simulink model "NFO"  (R2023a)
settings: Solver=FixedStepDiscrete  StartTime=0.0  StopTime=10  FixedStep=TsModel  RelTol=1e-3
values from neighbouring files (symbols this model uses):
  ADRC_times = 1.0    [NFO.sldd]
  b0 = 10000.0    [NFO.sldd]
  CCR_Counter = 8000.0    [NFO.sldd]
  current_bandwidth = 1500.0    [NFO.sldd]
  FLL_K = 1.414    [NFO.sldd]
  flux = 0.011    [NFO.sldd]
  Idq_limit = 20.0    [NFO.sldd]
  IF_Initial = 40.0    [NFO.sldd]
  Ls = 0.0001952    [NFO.sldd]
  Min_FLL_omega = 10.0    [NFO.sldd]
  omega_c = 50.0    [NFO.sldd]
  PLL_I = 3000.0    [NFO.sldd]
  PLL_P = 10.0    [NFO.sldd]
  PMSM_B = 0.0004924    [NFO.sldd]
  PMSM_J = 0.0027    [NFO.sldd]
  PMSM_Pn = 5.0    [NFO.sldd]
  Pn = 5.0    [NFO.sldd]
  Rs = 0.1763    [NFO.sldd]
  Swich_time = 1.5    [NFO.sldd]
  tao = -30.0    [NFO.sldd]
  Ts = 0.0001    [NFO.sldd]
  TsModel = 2.5E-5    [NFO.sldd]
undefined symbols (not defined in the file or in its folder): DiscIntNeverNeededParam, sigbuilder_block
libraries: slpidlib x3, mcbplantlib x1, autolibpmsmexterior x1
(part 1 of 2)
settings Model: DataDictionary=NFO.sldd  Creator=33595  LastModifiedBy=SkyLin
settings OptimizationCC: DefaultParameterBehavior=Inlined  UseDivisionForNetSlopeComputation=on  GainParamInheritBuiltInType=on  UseFloatMulNetSlope=on  InlineInvariantSignals=on  PassReuseOutputArgsAs=Individual arguments  ZeroExternalMemoryAtStartup=off  ZeroInternalMemoryAtStartup=off  NoFixptDivByZeroProtection=on  EfficientFloat2IntCast=on  LifeSpan=1  OptimizeBlockOrder=speed  DifferentSizesBufferReuse=on  EfficientTunableParamExpr=on
settings DebuggingCC: ParameterOverflowMsg=none  ParameterUnderflowMsg=error  ParameterPrecisionLossMsg=none  ParameterTunabilityLossMsg=error  UnconnectedInputMsg=warning  UnconnectedOutputMsg=warning  UnconnectedLineMsg=warning
settings HardwareCC: ProdBitPerPointer=32  ProdBitPerSizeT=32  ProdBitPerPtrDiffT=32  ProdLargestAtomicInteger=Long  ProdLargestAtomicFloat=Double  ProdWordSize=32  ProdLongLongMode=on  ProdHWDeviceType=ARM Compatible->ARM Cortex-M
settings ModelReferenceCC: EnableRefExpFcnMdlSchedulingChecks=on
settings SFSimCC: MATLABDynamicMemAlloc=off
settings RTWCC: Description=Embedded Coder  SystemTargetFile=ert.tlc  GenCodeOnly=on  TemplateMakefile=ert_default_tmf  RTWUseSimCustomCode=on  DLArmComputeVersion=19.05
settings CodeAppCC: ForceParamTrailComments=on  IgnoreCustomStorageClasses=off  OperatorAnnotations=on  SimulinkDataObjDesc=on  SFDataObjDesc=on  CustomSymbolStrGlobalVar=rt$N$M  CustomSymbolStrType=$N$M  CustomSymbolStrFcn=$N$M$F  CustomSymbolStrMacro=$N$M  InsertBlockDesc=on
settings ERTTargetCC: TargetLangStandard=C99 (ISO)  CodeReplacementLibrary=ARM Cortex-M  GenerateSampleERTMain=on  IncludeMdlTerminateFcn=off  CombineSignalStateStructs=on  SupportComplex=off  SupportNonInlinedSFcns=on  InlinedParameterPlacement=NonHierarchical  ERTCustomFileTemplate=example_file_process.tlc  ERTFilePackagingFormat=CompactWithDataFile  IndentSize=4

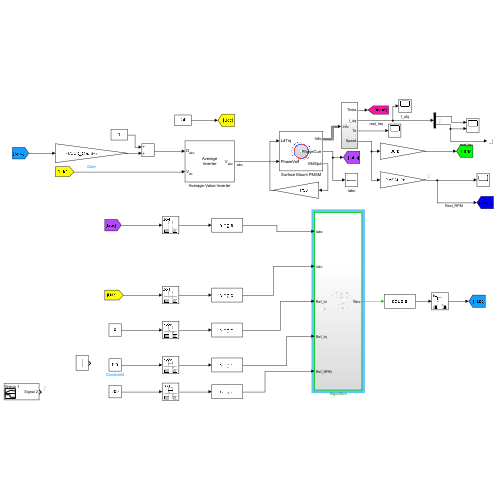
[thumbnail: Simulink's stored preview of the top-level diagram]
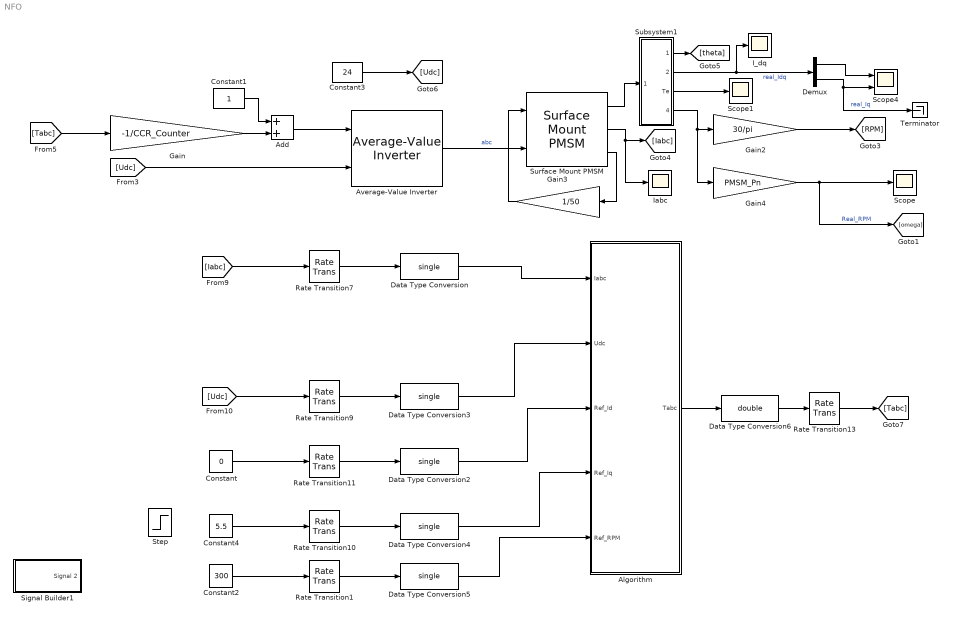
== system NFO ==
  Add : Sum
  Algorithm : Subsystem  TreatAsAtomicUnit=on
  Average-Value Inverter : mcbplantlib/Average-Value Inverter
  Constant : Constant  Value=0  OutDataTypeStr=single  SampleTime=Ts
  Constant1 : Constant  SampleTime=TsModel
  Constant2 : Constant  Value=300
  Constant3 : Constant  Value=24  SampleTime=TsModel
  Constant4 : Constant  Value=5.5  OutDataTypeStr=single  SampleTime=Ts
  Data Type Conversion{,2..5} (5 alike) : DataTypeConversion  OutDataTypeStr=single  SaturateOnIntegerOverflow=off  RndMeth=Floor
  Data Type Conversion6 : DataTypeConversion  OutDataTypeStr=double  SaturateOnIntegerOverflow=off  RndMeth=Floor
  Demux : Demux  Outputs=2
  Gain : Gain  Gain=-1/CCR_Counter
  Gain2 : Gain  Gain=30/pi
  Gain3 : Gain  Gain=1/50
  Gain4 : Gain  Gain=PMSM_Pn
  I_dq : Scope
  Iabc : Scope
  Rate Transition{1,9..11} (4 alike) : RateTransition  OutPortSampleTime=Ts
  Rate Transition13 : RateTransition  OutPortSampleTime=TsModel
  Rate Transition7 : RateTransition
  Scope : Scope
  Scope1 : Scope
  Scope4 : Scope  NumInputPorts=2
  Signal Builder1 : Subsystem  Tag=STV Subsys  LoadFcn=sigbuilder_block('load');  StartFcn=sigbuilder_block('start');  StopFcn=sigbuilder_block('stop');  ClipboardFcn=sigbuilder_block('clipboard');  mask(Sigbuilder block){tuvar=[0:10]}
      mask help: Simulink:masks:SigbuilderBlock_MD
      mask init:
      | if ~strcmp(get_param(bdroot(gcbh),'SimulationStatus'),'stopped') tuvar = sigbuilder_block('maskInit'); end
      settings: CopyFcn=sigbuilder_block('copy');  DeleteFcn=sigbuilder_block('delete');  ModelCloseFcn=sigbuilder_block('modelClose');  PreSaveFcn=sigbuilder_block('preSave');  PauseFcn=sigbuilder_block('pause');  ContinueFcn=sigbuilder_block('continue');  NameChangeFcn=sigbuilder_block('namechange');  OpenFcn=sigbuilder_block('open',[604 168 670.5 300 ]);  CloseFcn=sigbuilder_block('close');
      mask Display: plot(0, 0, 100, 100,[2, 2, 32, 32, 2], [68, 8, 8, 68, 68],[32, 2], [38, 38], [32, 19, 2],[53, 60, 44], [32, 17, 17, 2],[16, 16, 31, 31]);txt = getActiveGroup(gcbh);text(2, 100, txt,'verticalAlignment', 'top');
  Step : Step  Time=0  After=10  SampleTime=TsModel
  Subsystem1 : Subsystem
  Surface Mount PMSM : autolibpmsmexterior/Surface Mount PMSM  port_config=Torque  sim_type=Discrete  Ts=TsModel  P=PMSM_Pn  Rs=PMSM_Rs  Ldq_=PMSM_Ls  KConstText=Permanent flux linkage constant (lambda_pm):  lambda_pm=PMSM_flux  Ke=159.9771  Kt=1.323  mechanical=[PMSM_J, PMSM_B, 0]  idq0=[0 0]  theta_init=1  omega_init=0  KConst=PMSM_flux  lambda_pm_calc=PMSM_flux  RefBlkName='autolibpmsmexterior/Surface Mount PMSM'  aMode=5  Ldq="[0.0017      0.0017]"
  Terminator : Terminator
  wires:
  Constant3/1 -> [Udc]
  [Tabc] -> Gain/1
  Subsystem1/1(Theta) -> [theta]
  Subsystem1/2(I_dq) -> Demux/1, I_dq/1  "real_Idq"
  Subsystem1/3(Te) -> Scope1/1
  Subsystem1/4(Speed) -> Gain4/1, Gain2/1
  Average-Value Inverter/1 -> Surface Mount PMSM/2  "abc"
  Surface Mount PMSM/1 -> Subsystem1/1(Info)
  Surface Mount PMSM/2 -> Iabc/1, [Iabc]
  [Udc] -> Average-Value Inverter/2
  Gain2/1 -> [RPM]
  Surface Mount PMSM/3 -> Gain3/1
  Gain3/1 -> Surface Mount PMSM/1
  Gain4/1 -> [omega], Scope/1  "Real_RPM"
  Demux/2 -> Scope4/2, Terminator/1  "real_Iq"
  Data Type Conversion2/1 -> Algorithm/3(Ref_Id)
  [Udc] -> Rate Transition9/1
  Rate Transition13/1 -> [Tabc]
  [Iabc] -> Rate Transition7/1
  Rate Transition10/1 -> Data Type Conversion4/1
  Algorithm/1(Tabc) -> Data Type Conversion6/1
  Data Type Conversion/1 -> Algorithm/1(Iabc)
  Rate Transition11/1 -> Data Type Conversion2/1
  Rate Transition7/1 -> Data Type Conversion/1
  Data Type Conversion6/1 -> Rate Transition13/1
  Constant/1 -> Rate Transition11/1
  Data Type Conversion4/1 -> Algorithm/4(Ref_Iq)
  Rate Transition9/1 -> Data Type Conversion3/1
  Data Type Conversion3/1 -> Algorithm/2(Udc)
  Add/1 -> Average-Value Inverter/1
  Gain/1 -> Add/2
  Constant1/1 -> Add/1
  Demux/1 -> Scope4/1
  Rate Transition1/1 -> Data Type Conversion5/1
  Data Type Conversion5/1 -> Algorithm/5(Ref_RPM)
  Constant2/1 -> Rate Transition1/1
  Constant4/1 -> Rate Transition10/1

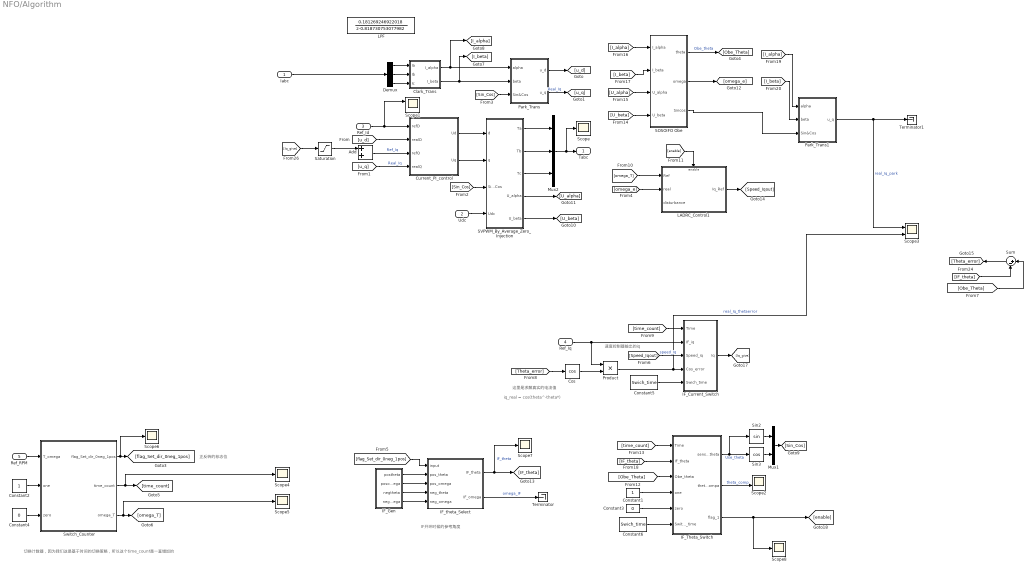
== system NFO/Algorithm ==
  note: iq_real = cos(theta^-theta*)
  note: 这里是求解真实的电流值
  note: 速度控制器输出的iq
  note: 正反转的标志位
  note: IF开环时候的参考角度
  note: 切换计数器，因为我们这是基于时间的切换策略，所以这个time_count是一直增加的
  Iabc : Inport  OutDataTypeStr=single
  Udc : Inport  Port=2  OutDataTypeStr=single
  Ref_Id : Inport  Port=3  OutDataTypeStr=single
  Ref_Iq : Inport  Port=4  OutDataTypeStr=single
  Ref_RPM : Inport  Port=5
  " Switch_Counter" : MATLAB Function  TreatAsAtomicUnit=on
  Add : Sum  OutDataTypeStr=single
  Clark_Trans : Subsystem  TreatAsAtomicUnit=on
      settings: RTWFcnNameOpts=Use subsystem name
  Constant1 : Constant  OutDataTypeStr=single
  Constant2 : Constant  OutDataTypeStr=single
  Constant3 : Constant  Value=0  OutDataTypeStr=single
  Constant4 : Constant  Value=0  OutDataTypeStr=single
  Constant5 : Constant  Value=Swich_time  OutDataTypeStr=single
  Constant6 : Constant  Value=Swich_time  OutDataTypeStr=single
  Cos : Trigonometry  Operator=cos
  Current_PI_control : Subsystem  TreatAsAtomicUnit=on
      settings: RTWFcnNameOpts=Use subsystem name
  Demux : Demux  Outputs=3
  IF_Current_Switch : MATLAB Function  TreatAsAtomicUnit=on
  IF_Gen : Subsystem
  IF_Theta_Switch : MATLAB Function  TreatAsAtomicUnit=on
  IF_theta_Select : MATLAB Function  TreatAsAtomicUnit=on
  LADRC_Control1 : Subsystem  TreatAsAtomicUnit=on
  LPF : DiscreteTransferFcn  Numerator=[0.181269246922018]  Denominator=[1 -0.818730753077982]
  Mux1 : Mux  Inputs=2
  Mux2 : Mux  Inputs=3
  Park_Trans : Subsystem  TreatAsAtomicUnit=on
      settings: RTWFcnNameOpts=Use subsystem name
  Park_Trans1 : Subsystem  TreatAsAtomicUnit=on
      settings: RTWFcnNameOpts=Use subsystem name
  Product : Product
  SOSOIFO Obe : Subsystem
  SVPWM_By_Average_Zero_Injection : Subsystem  TreatAsAtomicUnit=on
  Saturation : Saturate  UpperLimit=Idq_limit  LowerLimit=-Idq_limit  OutDataTypeStr=single
  Scope{,4..8} (6 alike) : Scope
  Scope1 : Scope  NumInputPorts=2
  Scope2 : Scope  NumInputPorts=2
  Scope3 : Scope  NumInputPorts=2
  Sin2 : Trigonometry
  Sin3 : Trigonometry  Operator=cos
  Sum : Sum  Inputs=|+-
  Terminator : Terminator
  Terminator1 : Terminator
  Tabc : Outport  OutDataTypeStr=single
  wires:
  Clark_Trans/2(I_beta) -> [I_beta], Park_Trans/2(beta)
  Clark_Trans/1(I_alpha) -> [I_alpha], Park_Trans/1(alpha)
  Demux/1 -> Clark_Trans/1(Ia)
  Demux/2 -> Clark_Trans/2(Ib)
  Demux/3 -> Clark_Trans/3(Ic)
  Park_Trans/1(u_d) -> [u_d]
  Park_Trans/2(u_q) -> [u_q]  "Real_Iq"
  Udc/1 -> SVPWM_By_Average_Zero_Injection/4(Udc)
  SVPWM_By_Average_Zero_Injection/1(Ta) -> Mux2/1
  SVPWM_By_Average_Zero_Injection/2(Tb) -> Mux2/2
  SVPWM_By_Average_Zero_Injection/3(Tc) -> Mux2/3
  SVPWM_By_Average_Zero_Injection/4(U_alpha) -> [U_alpha]
  SVPWM_By_Average_Zero_Injection/5(U_beta) -> [U_beta]
  [u_d] -> Current_PI_control/2(realD)
  [u_q] -> Current_PI_control/4(realQ)  "Real_Iq"
  Current_PI_control/1(Ud) -> SVPWM_By_Average_Zero_Injection/1(d)
  Current_PI_control/2(Uq) -> SVPWM_By_Average_Zero_Injection/2(q)
  [Sin_Cos] -> SVPWM_By_Average_Zero_Injection/3(Sin&Cos)
  [Sin_Cos] -> Park_Trans/3(Sin&Cos)
  Mux2/1 -> Tabc/1, Scope/1
  SOSOIFO Obe/1(theta) -> [Obe_Theta]  "Obe_theta"
  SOSOIFO Obe/2(omega) -> [omega_e]
  [I_alpha] -> SOSOIFO Obe/1(I_alpha)
  [U_alpha] -> SOSOIFO Obe/3(U_alpha)
  [I_beta] -> SOSOIFO Obe/2(I_beta)
  [U_beta] -> SOSOIFO Obe/4(U_beta)
  Ref_Id/1 -> Scope1/1, Current_PI_control/1(refD)
  [omega_e] -> LADRC_Control1/2(real)
  [omega_T] -> LADRC_Control1/1(Ref)
  Iabc/1 -> Demux/1
  Add/1 -> Current_PI_control/3(refQ)  "Ref_Iq"
  Constant2/1 -> " Switch_Counter"/2(one)
  Constant4/1 -> " Switch_Counter"/3(zero)
  Ref_RPM/1 -> " Switch_Counter"/1(T_omega)
  " Switch_Counter"/2(time_count) -> Scope4/1, [time_count]
  " Switch_Counter"/3(omega_T) -> Scope5/1, [omega_T]
  [Iq_give] -> Saturation/1
  Sum/1 -> [Theta_error]
  [Theta_error] -> Cos/1
  [Obe_Theta] -> Sum/1
  Constant3/1 -> IF_Theta_Switch/5(zero)
  IF_Theta_Switch/3(flag_1) -> Scope8/1, [enable]
  [IF_theta] -> Sum/2
  IF_Theta_Switch/1(sensorless_theta) -> Sin2/1, Sin3/1  "Use_theta"
  Sin3/1 -> Mux1/2
  Sin2/1 -> Mux1/1
  IF_Current_Switch/1(Iq) -> [Iq_give]
  Constant1/1 -> IF_Theta_Switch/4(one)
  LADRC_Control1/1(Iq_Ref) -> [Speed_Iqout]
  Ref_Iq/1 -> Product/1, IF_Current_Switch/2(IF_iq)
  [enable] -> LADRC_Control1/Enable
  " Switch_Counter"/1(flag_Set_dir_0neg_1pos) -> Scope6/1, [flag_Set_dir_0neg_1pos]
  Mux1/1 -> [Sin_Cos]
  Saturation/1 -> Add/1
  IF_Gen/1(postheta) -> IF_theta_Select/2(pos_theta)
  IF_Gen/2(posomega) -> IF_theta_Select/3(pos_omega)
  IF_Gen/3(negtheta) -> IF_theta_Select/4(neg_theta)
  IF_Gen/4(negomega) -> IF_theta_Select/5(neg_omega)
  [flag_Set_dir_0neg_1pos] -> IF_theta_Select/1(input)
  IF_theta_Select/1(IF_theta) -> Scope7/1, [IF_theta]  "IF_theta"
  [Obe_Theta] -> IF_Theta_Switch/3(Obe_theta)
  IF_Theta_Switch/2(theta_compa) -> Scope2/2  "theta_comp"
  [time_count] -> IF_Current_Switch/1(Time)
  [time_count] -> IF_Theta_Switch/1(Time)
  [Speed_Iqout] -> IF_Current_Switch/3(Speed_iq)  "speed_Iq"
  Product/1 -> Scope3/2, IF_Current_Switch/4(Cos_error)  "real_Iq_thetaerror"
  Cos/1 -> Product/2
  Constant5/1 -> IF_Current_Switch/5(Swich_time)
  IF_theta_Select/2(IF_omega) -> Terminator/1  "omega_IF"
  Constant6/1 -> IF_Theta_Switch/6(Switch_time)
  [IF_theta] -> IF_Theta_Switch/2(IF_theta)
  SOSOIFO Obe/3(Sincos) -> Park_Trans1/3(Sin&Cos)
  [I_beta] -> Park_Trans1/2(beta)
  [I_alpha] -> Park_Trans1/1(alpha)
  Park_Trans1/1(u_q) -> Scope3/1, Terminator1/1  "real_Iq_park"

== system NFO/Signal Builder1 ==
  Demux : Demux  Tag=STV Demux  Outputs=1
      settings: DisplayOption=none
  FromWs : FromWorkspace  Tag=STV FromWs  VariableName=tuvar
      SigBuilderData=|
      | common.afterFinalStr = 'Extrapolate'
      | common.sampleTime = 0
      | dataSet.timeRange = [0 10]
      | dataSet.name = 'Group 1'
      | sbobj.Groups.Name = 'Group 1'
      | sbobj.Groups.Signals.Name = 'Signal 2'
      | sbobj.Groups.Signals.XData = [0 5.72 5.72 10]
      | sbobj.Groups.Signals.YData = [126 126 234 234]
  Signal 2 : Outport  Tag=STV Outport
  wires:
  Demux/1 -> Signal 2/1
  FromWs/1 -> Demux/1

== system NFO/Subsystem1 ==
  Info : Inport
  Bus Selector2 : BusSelector  OutputSignals=IdSync,IqSync,MtrPos,MtrTrq,MtrSpd
  Constant4 : Constant  Value=2*pi  SampleTime=-1
  Gain2 : Gain  Gain=Pn
  Mod1 : Math  Operator=mod
  Mux : Mux  Inputs=2
  Scope : Scope
  Theta : Outport
  I_dq : Outport  Port=2
  Te : Outport  Port=3
  Speed : Outport  Port=4
  wires:
  Bus Selector2/2 -> Mux/2  "<IqSync>"
  Gain2/1 -> Mod1/1
  Mod1/1 -> Theta/1
  Bus Selector2/1 -> Mux/1  "<IdSync>"
  Constant4/1 -> Mod1/2
  Info/1 -> Bus Selector2/1
  Bus Selector2/3 -> Gain2/1  "<MtrPos>"
  Mux/1 -> I_dq/1
  Bus Selector2/4 -> Te/1  "<MtrTrq>"
  Bus Selector2/5 -> Scope/1, Speed/1  "<MtrSpd>"

== system NFO/Algorithm/Clark_Trans ==
  note: $u_\alpha=\frac{2}{3}(u_a-\frac{1}{2}u_b-\frac{1}{2}u_c ) \\ u_\beta=\frac{2}{3}(\frac{\sqrt{3}}{2}u_b-\frac{\sqrt{3}}{2}u_c)$
  note: Clark_Transform
  Ia : Inport  OutDataTypeStr=single
  Ib : Inport  Port=2  OutDataTypeStr=single
  Ic : Inport  Port=3  OutDataTypeStr=single
  Add : Sum  Inputs=+-  OutDataTypeStr=single
  Add1 : Sum  OutDataTypeStr=single
  Add2 : Sum  Inputs=+-  OutDataTypeStr=single
  Gain : Gain  Gain=0.5  OutDataTypeStr=single
  Gain1 : Gain  Gain=single(sqrt(3)/3)  OutDataTypeStr=single
  Gain2 : Gain  Gain=single(2/3)  OutDataTypeStr=single
  I_alpha : Outport  OutDataTypeStr=single
  I_beta : Outport  Port=2
  wires:
  Ia/1 -> Add/1
  Gain/1 -> Add/2
  Ib/1 -> Add1/1, Add2/1
  Ic/1 -> Add1/2, Add2/2
  Add2/1 -> Gain1/1
  Add1/1 -> Gain/1
  Add/1 -> Gain2/1
  Gain2/1 -> I_alpha/1
  Gain1/1 -> I_beta/1

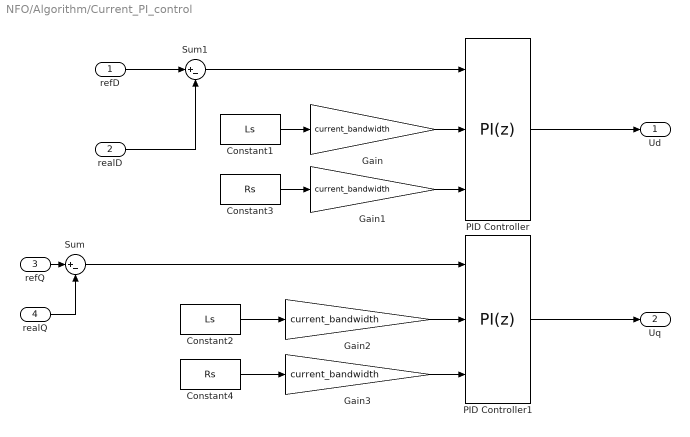
== system NFO/Algorithm/Current_PI_control ==
  refD : Inport  OutDataTypeStr=single
  realD : Inport  Port=2  OutDataTypeStr=single
  refQ : Inport  Port=3  OutDataTypeStr=single
  realQ : Inport  Port=4  OutDataTypeStr=single
  Constant1 : Constant  Value=Ls  OutDataTypeStr=single  SampleTime=Ts
  Constant2 : Constant  Value=Ls  OutDataTypeStr=single  SampleTime=Ts
  Constant3 : Constant  Value=Rs  OutDataTypeStr=single  SampleTime=Ts
  Constant4 : Constant  Value=Rs  OutDataTypeStr=single  SampleTime=Ts
  Gain{,1..3} (4 alike) : Gain  Gain=current_bandwidth  OutDataTypeStr=single
  PID Controller : slpidlib/PID Controller  Controller=PI  Form=Parallel  TimeDomain=Discrete-time  UseExternalTs=off  SampleTime=Ts  IntegratorMethod=Forward Euler  FilterMethod=Forward Euler  ControllerParametersSource=external  P=1  I=1  UseKiTs=off  D=0  N=100  UseFilter=on  TunerSelectOption=Transfer Function Based (PID Tuner App)  ZeroCross=off  InitialConditionSource=internal  InitialConditionForIntegrator=0  InitialConditionForFilter=0  DifferentiatorICPrevScaledInput=0  ExternalReset=none  TrackingMode=off  Kt=1  LimitOutput=on  SatLimitsSource=internal  UpperSaturationLimit=Idq_limit  LowerSaturationLimit=-Idq_limit  LinearizeAsGain=off  AntiWindupMode=none  Kb=1  LimitIntegrator=off  UpperIntegratorSaturationLimit=inf  LowerIntegratorSaturationLimit=-inf  POutMin=[]  POutMax=[]  IOutMin=[]  IOutMax=[]  DOutMin=[]  DOutMax=[]  NOutMin=[]  NOutMax=[]  SumOutMin=[]  SumOutMax=[]  SaturationOutMin=[]  SaturationOutMax=[]  PParamMin=[]  PParamMax=[]  IParamMin=[]  IParamMax=[]  DParamMin=[]  DParamMax=[]  NParamMin=[]  NParamMax=[]  KbParamMin=[]  KbParamMax=[]  KtParamMin=[]  KtParamMax=[]  KbOutMin=[]  KbOutMax=[]  KtOutMin=[]  KtOutMax=[]  IntegratorOutMin=[]  IntegratorOutMax=[]  FilterOutMin=[]  FilterOutMax=[]  SumI1OutMin=[]  SumI1OutMax=[]  SumI2OutMin=[]  SumI2OutMax=[]  SumI3OutMin=[]  SumI3OutMax=[]  SumI4OutMin=[]  SumI4OutMax=[]  SumDOutMin=[]  SumDOutMax=[]  DifferentiatorOutMin=[]  DifferentiatorOutMax=[]  FilterDiffOutCoefMin=[]  FilterDiffOutCoefMax=[]  ReciprocalOutMin=[]  ReciprocalOutMax=[]  SumDenOutMin=[]  SumDenOutMax=[]  SumNumOutMin=[]  SumNumOutMax=[]  DivideOutMin=[]  DivideOutMax=[]  UdiffTsProdOutMin=[]  UdiffTsProdOutMax=[]  NTsProdOutMin=[]  NTsProdOutMax=[]  UintegralTsProdOutMin=[]  UintegralTsProdOutMax=[]  UngainTsProdOutMin=[]  UngainTsProdOutMax=[]  ClampingZeroOutDataTypeStr=Inherit: Inherit via back propagation  ClampingZeroOutMin=[]  ClampingZeroOutMax=[]  FilterDenConstantOutDataTypeStr=Inherit: Inherit via back propagation  FilterDenConstantOutMin=[]  FilterDenConstantOutMax=[]  PCopyOutDataTypeStr=Inherit: Inherit via back propagation  PCopyOutMin=[]  PCopyOutMax=[]  NCopyOutDataTypeStr=Inherit: Inherit via back propagation  NCopyOutMin=[]  NCopyOutMax=[]  IntegratorContinuousStateAttributes=''  IntegratorStateMustResolveToSignalObject=off  IntegratorRTWStateStorageClass=Auto  FilterContinuousStateAttributes=''  FilterStateMustResolveToSignalObject=off  FilterRTWStateStorageClass=Auto  ParallelPVariant=ExternalParameters  IdealPVariant=Disabled  IVariant=ExternalParameters  DVariant=Disabled  IntegratorVariant=Discrete  SatVariant=Enabled  AWVariant=Passthrough  PCopyVariant=Disabled  TRVariant=Disabled  FdbkBlocksVariant=Forward  IdealPFdbkVariant=Disabled  SatFdbkVariant=Disabled  DerivativeFilterVariant=Disabled  NVariant=Disabled  NCopyVariant=Disabled_SignalSpec  FilterICVariant=Disabled  IntegratorICVariant=InternalICs  ExternalResetVariant=Disabled  TRSumVariant=Passthrough  SumFdbkVariant=Disabled  SumVariant=Sum_PI  TsampFilterVariant=InternalTs  TsampNgainVariant=Passthrough  TsampIntegralVariant=Disabled_SignalSpec  ExternalSaturationOutDataTypeStr=Inherit: Same as second input
  PID Controller1 : slpidlib/PID Controller  Controller=PI  Form=Parallel  TimeDomain=Discrete-time  UseExternalTs=off  SampleTime=Ts  IntegratorMethod=Forward Euler  FilterMethod=Forward Euler  ControllerParametersSource=external  P=1  I=1  UseKiTs=off  D=0  N=100  UseFilter=on  TunerSelectOption=Transfer Function Based (PID Tuner App)  ZeroCross=off  InitialConditionSource=internal  InitialConditionForIntegrator=0  InitialConditionForFilter=0  DifferentiatorICPrevScaledInput=0  ExternalReset=none  TrackingMode=off  Kt=1  LimitOutput=on  SatLimitsSource=internal  UpperSaturationLimit=Idq_limit  LowerSaturationLimit=-Idq_limit  LinearizeAsGain=off  AntiWindupMode=none  Kb=1  LimitIntegrator=off  UpperIntegratorSaturationLimit=inf  LowerIntegratorSaturationLimit=-inf  POutMin=[]  POutMax=[]  IOutMin=[]  IOutMax=[]  DOutMin=[]  DOutMax=[]  NOutMin=[]  NOutMax=[]  SumOutMin=[]  SumOutMax=[]  SaturationOutMin=[]  SaturationOutMax=[]  PParamMin=[]  PParamMax=[]  IParamMin=[]  IParamMax=[]  DParamMin=[]  DParamMax=[]  NParamMin=[]  NParamMax=[]  KbParamMin=[]  KbParamMax=[]  KtParamMin=[]  KtParamMax=[]  KbOutMin=[]  KbOutMax=[]  KtOutMin=[]  KtOutMax=[]  IntegratorOutMin=[]  IntegratorOutMax=[]  FilterOutMin=[]  FilterOutMax=[]  SumI1OutMin=[]  SumI1OutMax=[]  SumI2OutMin=[]  SumI2OutMax=[]  SumI3OutMin=[]  SumI3OutMax=[]  SumI4OutMin=[]  SumI4OutMax=[]  SumDOutMin=[]  SumDOutMax=[]  DifferentiatorOutMin=[]  DifferentiatorOutMax=[]  FilterDiffOutCoefMin=[]  FilterDiffOutCoefMax=[]  ReciprocalOutMin=[]  ReciprocalOutMax=[]  SumDenOutMin=[]  SumDenOutMax=[]  SumNumOutMin=[]  SumNumOutMax=[]  DivideOutMin=[]  DivideOutMax=[]  UdiffTsProdOutMin=[]  UdiffTsProdOutMax=[]  NTsProdOutMin=[]  NTsProdOutMax=[]  UintegralTsProdOutMin=[]  UintegralTsProdOutMax=[]  UngainTsProdOutMin=[]  UngainTsProdOutMax=[]  ClampingZeroOutDataTypeStr=Inherit: Inherit via back propagation  ClampingZeroOutMin=[]  ClampingZeroOutMax=[]  FilterDenConstantOutDataTypeStr=Inherit: Inherit via back propagation  FilterDenConstantOutMin=[]  FilterDenConstantOutMax=[]  PCopyOutDataTypeStr=Inherit: Inherit via back propagation  PCopyOutMin=[]  PCopyOutMax=[]  NCopyOutDataTypeStr=Inherit: Inherit via back propagation  NCopyOutMin=[]  NCopyOutMax=[]  IntegratorContinuousStateAttributes=''  IntegratorStateMustResolveToSignalObject=off  IntegratorRTWStateStorageClass=Auto  FilterContinuousStateAttributes=''  FilterStateMustResolveToSignalObject=off  FilterRTWStateStorageClass=Auto  ParallelPVariant=ExternalParameters  IdealPVariant=Disabled  IVariant=ExternalParameters  DVariant=Disabled  IntegratorVariant=Discrete  SatVariant=Enabled  AWVariant=Passthrough  PCopyVariant=Disabled  TRVariant=Disabled  FdbkBlocksVariant=Forward  IdealPFdbkVariant=Disabled  SatFdbkVariant=Disabled  DerivativeFilterVariant=Disabled  NVariant=Disabled  NCopyVariant=Disabled_SignalSpec  FilterICVariant=Disabled  IntegratorICVariant=InternalICs  ExternalResetVariant=Disabled  TRSumVariant=Passthrough  SumFdbkVariant=Disabled  SumVariant=Sum_PI  TsampFilterVariant=InternalTs  TsampNgainVariant=Passthrough  TsampIntegralVariant=Disabled_SignalSpec  ExternalSaturationOutDataTypeStr=Inherit: Same as second input
  Sum : Sum  Inputs=|+-  OutDataTypeStr=single
  Sum1 : Sum  Inputs=|+-  OutDataTypeStr=single
  Ud : Outport  OutDataTypeStr=single
  Uq : Outport  Port=2  OutDataTypeStr=single
  wires:
  realD/1 -> Sum1/2
  realQ/1 -> Sum/2
  PID Controller1/1 -> Uq/1
  PID Controller/1 -> Ud/1
  Sum/1 -> PID Controller1/1
  Sum1/1 -> PID Controller/1
  refD/1 -> Sum1/1
  refQ/1 -> Sum/1
  Constant2/1 -> Gain2/1
  Gain3/1 -> PID Controller1/3
  Gain/1 -> PID Controller/2
  Gain2/1 -> PID Controller1/2
  Constant1/1 -> Gain/1
  Constant4/1 -> Gain3/1
  Gain1/1 -> PID Controller/3
  Constant3/1 -> Gain1/1

== system NFO/Algorithm/IF_Gen ==
  IFneg : Subsystem  TreatAsAtomicUnit=on
      mask Display:
      | port_label('output',1,'negtheta','texmode','on');
      | port_label('output',2,'negomega','texmode','on');
      | 
      | fprintf('IFneg_theta');
  IFpos : Subsystem  TreatAsAtomicUnit=on
      mask Display:
      | port_label('output',1,'postheta','texmode','on');
      | port_label('output',2,'posomega','texmode','on');
      | 
      | fprintf('IFpos_theta');
  postheta : Outport
  posomega : Outport  Port=2
  negtheta : Outport  Port=3
  negomega : Outport  Port=4
  wires:
  IFpos/1(theta) -> postheta/1
  IFneg/2(omega) -> negomega/1
  IFneg/1(theta) -> negtheta/1
  IFpos/2(omega) -> posomega/1

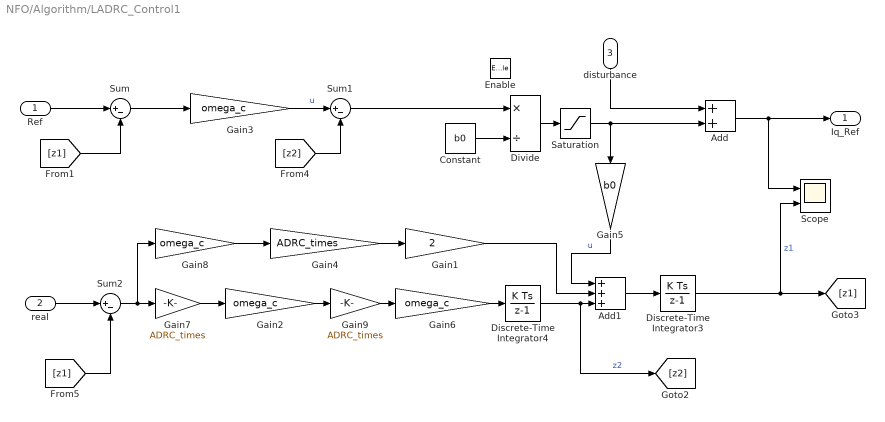
== system NFO/Algorithm/LADRC_Control1 ==
  Ref : Inport  OutDataTypeStr=single
  real : Inport  Port=2  OutDataTypeStr=single
  disturbance : Inport  Port=3  OutDataTypeStr=single
  Enable : EnablePort
  Add : Sum  OutDataTypeStr=single
  Add1 : Sum  Inputs=+++  OutDataTypeStr=single
  Constant : Constant  Value=b0  OutDataTypeStr=single
  Discrete-Time Integrator3 : DiscreteIntegrator  SampleTime=-1  OutDataTypeStr=single  LimitOutput=on  UpperSaturationLimit=2500  LowerSaturationLimit=-2500  ICPrevOutput=DiscIntNeverNeededParam  ICPrevScaledInput=DiscIntNeverNeededParam
  Discrete-Time Integrator4 : DiscreteIntegrator  SampleTime=-1  OutDataTypeStr=single  ICPrevOutput=DiscIntNeverNeededParam  ICPrevScaledInput=DiscIntNeverNeededParam
  Divide : Product  Inputs=*/  OutDataTypeStr=single
  Gain1 : Gain  Gain=2  OutDataTypeStr=single
  Gain{2..3,6,8} (4 alike) : Gain  Gain=omega_c  OutDataTypeStr=single
  Gain4 : Gain  Gain=ADRC_times  OutDataTypeStr=single
  Gain5 : Gain  Gain=b0  OutDataTypeStr=single
  Gain7 : Gain  Gain=ADRC_times  OutDataTypeStr=single
  Gain9 : Gain  Gain=ADRC_times  OutDataTypeStr=single
  Saturation : Saturate  UpperLimit=Idq_limit  LowerLimit=-Idq_limit  OutDataTypeStr=single
  Scope : Scope  NumInputPorts=2
  Sum : Sum  Inputs=|+-  OutDataTypeStr=single
  Sum1 : Sum  Inputs=|+-  OutDataTypeStr=single
  Sum2 : Sum  Inputs=|+-  OutDataTypeStr=single
  Iq_Ref : Outport  OutDataTypeStr=single
  wires:
  Ref/1 -> Sum/1
  Discrete-Time Integrator4/1 -> Add1/3, [z2]  "z2"
  Gain5/1 -> Add1/1  "u"
  Gain2/1 -> Gain9/1
  Gain1/1 -> Add1/2
  Discrete-Time Integrator3/1 -> Scope/2, [z1]  "z1"
  Add1/1 -> Discrete-Time Integrator3/1
  Sum2/1 -> Gain7/1, Gain8/1
  real/1 -> Sum2/1
  [z1] -> Sum2/2
  [z1] -> Sum/2
  Sum/1 -> Gain3/1
  [z2] -> Sum1/2
  Constant/1 -> Divide/2
  Divide/1 -> Saturation/1
  Gain3/1 -> Sum1/1  "u"
  Sum1/1 -> Divide/1
  Add/1 -> Scope/1, Iq_Ref/1
  disturbance/1 -> Add/1
  Saturation/1 -> Add/2, Gain5/1
  Gain4/1 -> Gain1/1
  Gain6/1 -> Discrete-Time Integrator4/1
  Gain7/1 -> Gain2/1
  Gain8/1 -> Gain4/1
  Gain9/1 -> Gain6/1

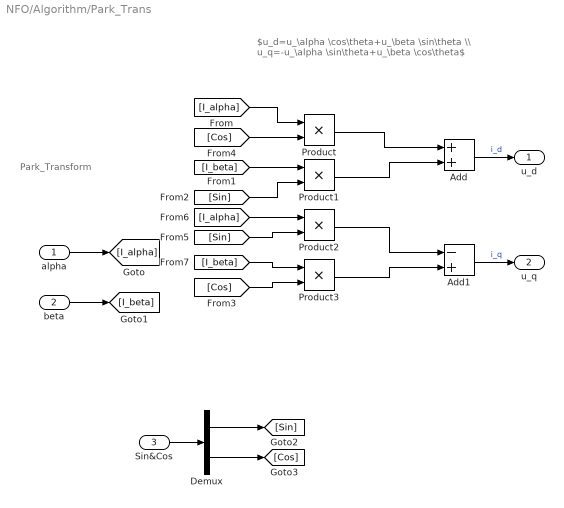
== system NFO/Algorithm/Park_Trans ==
  note: $u_d=u_\alpha \cos\theta+u_\beta \sin\theta \\ u_q=-u_\alpha \sin\theta+u_\beta \cos\theta$
  note: Park_Transform
  alpha : Inport  OutDataTypeStr=single
  beta : Inport  Port=2  OutDataTypeStr=single
  Sin&Cos : Inport  Port=3  OutDataTypeStr=single
  Add : Sum  OutDataTypeStr=single
  Add1 : Sum  Inputs=-+  OutDataTypeStr=single
  Demux : Demux  Outputs=2
  Product{,1..3} (4 alike) : Product  OutDataTypeStr=single
  u_d : Outport  OutDataTypeStr=single
  u_q : Outport  Port=2  OutDataTypeStr=single
  wires:
  Add1/1 -> u_q/1  "i_q"
  [Cos] -> Product/2
  Product/1 -> Add/1
  Product1/1 -> Add/2
  beta/1 -> [I_beta]
  Add/1 -> u_d/1  "i_d"
  [I_alpha] -> Product/1
  Product3/1 -> Add1/2
  [I_beta] -> Product3/1
  [I_beta] -> Product1/1
  [Sin] -> Product2/2
  Product2/1 -> Add1/1
  [Sin] -> Product1/2
  [I_alpha] -> Product2/1
  alpha/1 -> [I_alpha]
  [Cos] -> Product3/2
  Demux/1 -> [Sin]
  Demux/2 -> [Cos]
  Sin&Cos/1 -> Demux/1

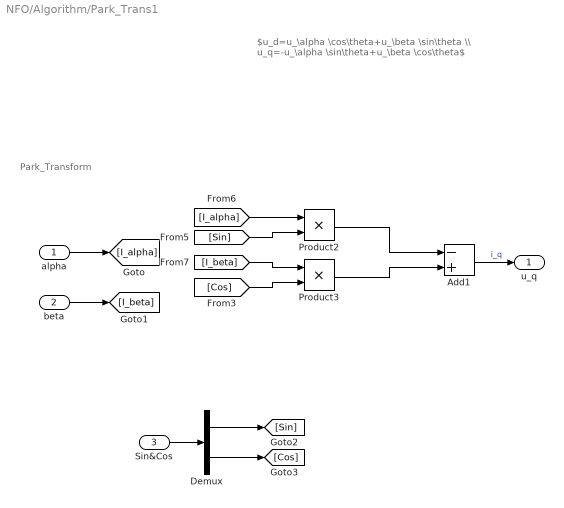
== system NFO/Algorithm/Park_Trans1 ==
  note: $u_d=u_\alpha \cos\theta+u_\beta \sin\theta \\ u_q=-u_\alpha \sin\theta+u_\beta \cos\theta$
  note: Park_Transform
  alpha : Inport  OutDataTypeStr=single
  beta : Inport  Port=2  OutDataTypeStr=single
  Sin&Cos : Inport  Port=3  OutDataTypeStr=single
  Add1 : Sum  Inputs=-+  OutDataTypeStr=single
  Demux : Demux  Outputs=2
  Product2 : Product  OutDataTypeStr=single
  Product3 : Product  OutDataTypeStr=single
  u_q : Outport  OutDataTypeStr=single
  wires:
  Add1/1 -> u_q/1  "i_q"
  beta/1 -> [I_beta]
  Product3/1 -> Add1/2
  [I_beta] -> Product3/1
  [Sin] -> Product2/2
  Product2/1 -> Add1/1
  [I_alpha] -> Product2/1
  alpha/1 -> [I_alpha]
  [Cos] -> Product3/2
  Demux/1 -> [Sin]
  Demux/2 -> [Cos]
  Sin&Cos/1 -> Demux/1

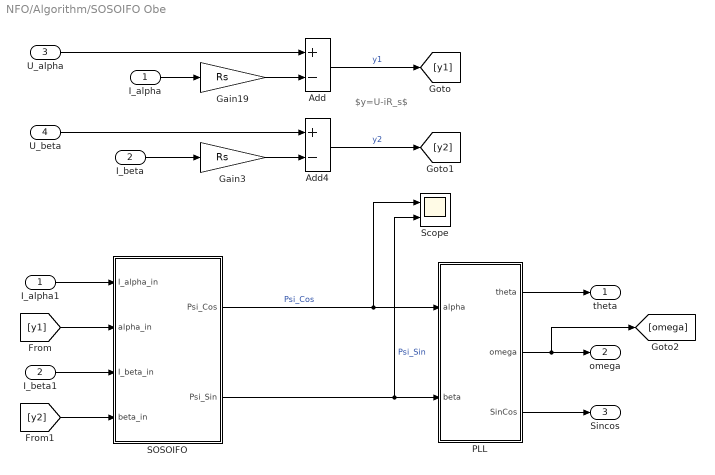
== system NFO/Algorithm/SOSOIFO Obe ==
  note: $y=U-iR_s$
  I_alpha : Inport  OutDataTypeStr=single
  I_beta : Inport  Port=2  OutDataTypeStr=single
  U_alpha : Inport  Port=3  OutDataTypeStr=single
  U_beta : Inport  Port=4  OutDataTypeStr=single
  Add : Sum  Inputs=+-  OutDataTypeStr=single
  Add4 : Sum  Inputs=+-  OutDataTypeStr=single
  Gain19 : Gain  Gain=Rs  OutDataTypeStr=single
  Gain3 : Gain  Gain=Rs  OutDataTypeStr=single
  I_alpha1 : InportShadow  OutDataTypeStr=single
  I_beta1 : InportShadow  Port=2  OutDataTypeStr=single
  PLL : Subsystem
  SOSOIFO : Subsystem
  Scope : Scope  NumInputPorts=2
  theta : Outport  OutDataTypeStr=single
  omega : Outport  Port=2  OutDataTypeStr=single
  Sincos : Outport  Port=3  OutDataTypeStr=single
  wires:
  PLL/1(theta) -> theta/1
  PLL/2(omega) -> [omega], omega/1
  Add4/1 -> [y2]  "y2"
  U_alpha/1 -> Add/1
  Add/1 -> [y1]  "y1"
  U_beta/1 -> Add4/1
  I_alpha/1 -> Gain19/1
  I_beta/1 -> Gain3/1
  SOSOIFO/1(Psi_Cos) -> PLL/1(alpha), Scope/1  "Psi_Cos"
  SOSOIFO/2(Psi_Sin) -> Scope/2, PLL/2(beta)  "Psi_Sin"
  PLL/3(SinCos) -> Sincos/1
  Gain19/1 -> Add/2
  Gain3/1 -> Add4/2
  [y1] -> SOSOIFO/2(alpha_in)
  [y2] -> SOSOIFO/4(beta_in)
  I_beta1/1 -> SOSOIFO/3(I_beta_in)
  I_alpha1/1 -> SOSOIFO/1(I_alpha_in)

== system NFO/Algorithm/SVPWM_By_Average_Zero_Injection ==
  d : Inport  OutDataTypeStr=single
  q : Inport  Port=2  OutDataTypeStr=single
  Sin&Cos : Inport  Port=3  OutDataTypeStr=single
  Udc : Inport  Port=4  OutDataTypeStr=single
  Anti_Park_Trans : Subsystem
  SVPWM : Subsystem
  Ta : Outport  OutDataTypeStr=single
  Tb : Outport  Port=2  OutDataTypeStr=single
  Tc : Outport  Port=3  OutDataTypeStr=single
  U_alpha : Outport  Port=4  OutDataTypeStr=single
  U_beta : Outport  Port=5  OutDataTypeStr=single
  wires:
  Anti_Park_Trans/1(alpha) -> U_alpha/1, SVPWM/1(alpha)
  q/1 -> Anti_Park_Trans/2(q)
  Anti_Park_Trans/2(beta) -> U_beta/1, SVPWM/2(beta)
  d/1 -> Anti_Park_Trans/1(d)
  Sin&Cos/1 -> Anti_Park_Trans/3(Sin&Cos)
  Udc/1 -> SVPWM/3(Udc)
  SVPWM/1(Ta) -> Ta/1
  SVPWM/2(Tb) -> Tb/1
  SVPWM/3(Tc) -> Tc/1

== system NFO/Algorithm/IF_Gen/IFneg ==
  Constant : Constant  Value=IF_Initial  OutDataTypeStr=single
  Discrete-Time Integrator : DiscreteIntegrator  SampleTime=-1  ICPrevOutput=DiscIntNeverNeededParam  ICPrevScaledInput=DiscIntNeverNeededParam
  Gain : Gain  Gain=-1
  integrator : Subsystem
  theta : Outport  OutDataTypeStr=single
  omega : Outport  Port=2  OutDataTypeStr=single
  wires:
  integrator/1(y(k-1)) -> theta/1
  Constant/1 -> Gain/1
  Gain/1 -> Discrete-Time Integrator/1
  Discrete-Time Integrator/1 -> omega/1, integrator/1(x(k))

== system NFO/Algorithm/IF_Gen/IFpos ==
  Constant : Constant  Value=IF_Initial  OutDataTypeStr=single
  Discrete-Time Integrator : DiscreteIntegrator  SampleTime=-1  ICPrevOutput=DiscIntNeverNeededParam  ICPrevScaledInput=DiscIntNeverNeededParam
  Scope : Scope
  Scope1 : Scope
  integrator : Subsystem
  theta : Outport  OutDataTypeStr=single
  omega : Outport  Port=2  OutDataTypeStr=single
  wires:
  integrator/1(y(k-1)) -> Scope1/1, theta/1
  Constant/1 -> Discrete-Time Integrator/1
  Discrete-Time Integrator/1 -> Scope/1, omega/1, integrator/1(x(k))

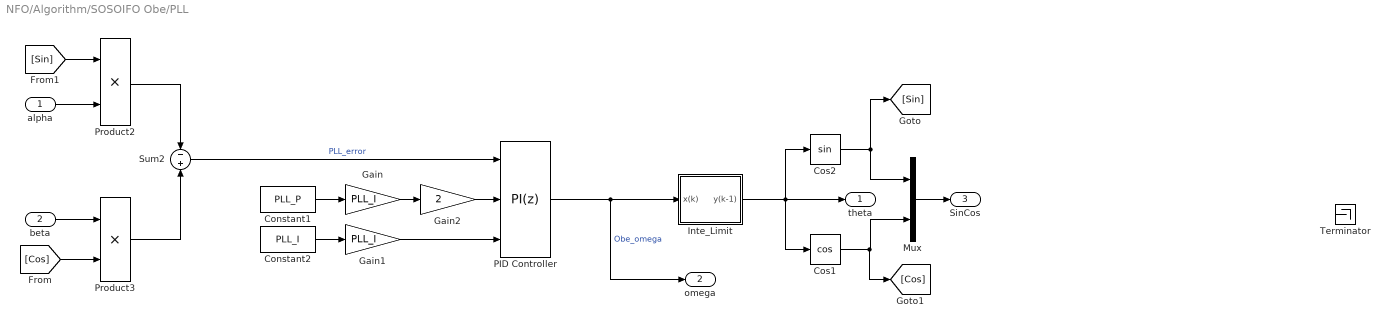
== system NFO/Algorithm/SOSOIFO Obe/PLL ==
  alpha : Inport  OutDataTypeStr=single
  beta : Inport  Port=2  OutDataTypeStr=single
  Constant1 : Constant  Value=PLL_P  OutDataTypeStr=single
  Constant2 : Constant  Value=PLL_I  OutDataTypeStr=single
  Cos1 : Trigonometry  Operator=cos
  Cos2 : Trigonometry
  Gain : Gain  Gain=PLL_I
  Gain1 : Gain  Gain=PLL_I
  Gain2 : Gain  Gain=2
  Inte_Limit : Subsystem
  Mux : Mux  Inputs=2
  PID Controller : slpidlib/PID Controller  Controller=PI  Form=Parallel  TimeDomain=Discrete-time  UseExternalTs=off  SampleTime=Ts  IntegratorMethod=Forward Euler  FilterMethod=Forward Euler  ControllerParametersSource=external  P=2*PLL_P*PLL_I  I=PLL_I*PLL_I  UseKiTs=off  D=0  N=100  UseFilter=on  TunerSelectOption=Transfer Function Based (PID Tuner App)  ZeroCross=off  InitialConditionSource=internal  InitialConditionForIntegrator=0  InitialConditionForFilter=0  DifferentiatorICPrevScaledInput=0  ExternalReset=none  TrackingMode=off  Kt=1  LimitOutput=on  SatLimitsSource=internal  UpperSaturationLimit=1400  LowerSaturationLimit=-1400  LinearizeAsGain=on  AntiWindupMode=none  Kb=1  LimitIntegrator=off  UpperIntegratorSaturationLimit=inf  LowerIntegratorSaturationLimit=-inf  POutMin=[]  POutMax=[]  IOutMin=[]  IOutMax=[]  DOutMin=[]  DOutMax=[]  NOutMin=[]  NOutMax=[]  SumOutMin=[]  SumOutMax=[]  SaturationOutMin=[]  SaturationOutMax=[]  PParamMin=[]  PParamMax=[]  IParamMin=[]  IParamMax=[]  DParamMin=[]  DParamMax=[]  NParamMin=[]  NParamMax=[]  KbParamMin=[]  KbParamMax=[]  KtParamMin=[]  KtParamMax=[]  KbOutMin=[]  KbOutMax=[]  KtOutMin=[]  KtOutMax=[]  IntegratorOutMin=[]  IntegratorOutMax=[]  FilterOutMin=[]  FilterOutMax=[]  SumI1OutMin=[]  SumI1OutMax=[]  SumI2OutMin=[]  SumI2OutMax=[]  SumI3OutMin=[]  SumI3OutMax=[]  SumI4OutMin=[]  SumI4OutMax=[]  SumDOutMin=[]  SumDOutMax=[]  DifferentiatorOutMin=[]  DifferentiatorOutMax=[]  FilterDiffOutCoefMin=[]  FilterDiffOutCoefMax=[]  ReciprocalOutMin=[]  ReciprocalOutMax=[]  SumDenOutMin=[]  SumDenOutMax=[]  SumNumOutMin=[]  SumNumOutMax=[]  DivideOutMin=[]  DivideOutMax=[]  UdiffTsProdOutMin=[]  UdiffTsProdOutMax=[]  NTsProdOutMin=[]  NTsProdOutMax=[]  UintegralTsProdOutMin=[]  UintegralTsProdOutMax=[]  UngainTsProdOutMin=[]  UngainTsProdOutMax=[]  ClampingZeroOutDataTypeStr=Inherit: Inherit via back propagation  ClampingZeroOutMin=[]  ClampingZeroOutMax=[]  FilterDenConstantOutDataTypeStr=Inherit: Inherit via back propagation  FilterDenConstantOutMin=[]  FilterDenConstantOutMax=[]  PCopyOutDataTypeStr=Inherit: Inherit via back propagation  PCopyOutMin=[]  PCopyOutMax=[]  NCopyOutDataTypeStr=Inherit: Inherit via back propagation  NCopyOutMin=[]  NCopyOutMax=[]  IntegratorContinuousStateAttributes=''  IntegratorStateMustResolveToSignalObject=off  IntegratorRTWStateStorageClass=Auto  FilterContinuousStateAttributes=''  FilterStateMustResolveToSignalObject=off  FilterRTWStateStorageClass=Auto  ParallelPVariant=ExternalParameters  IdealPVariant=Disabled  IVariant=ExternalParameters  DVariant=Disabled  IntegratorVariant=Discrete  SatVariant=Enabled  AWVariant=Passthrough  PCopyVariant=Disabled  TRVariant=Disabled  FdbkBlocksVariant=Forward  IdealPFdbkVariant=Disabled  SatFdbkVariant=Disabled  DerivativeFilterVariant=Disabled  NVariant=Disabled  NCopyVariant=Disabled_SignalSpec  FilterICVariant=Disabled  IntegratorICVariant=InternalICs  ExternalResetVariant=Disabled  TRSumVariant=Passthrough  SumFdbkVariant=Disabled  SumVariant=Sum_PI  TsampFilterVariant=InternalTs  TsampNgainVariant=Passthrough  TsampIntegralVariant=Disabled_SignalSpec  ExternalSaturationOutDataTypeStr=Inherit: Same as second input
  Product2 : Product  OutDataTypeStr=single
  Product3 : Product  OutDataTypeStr=single
  Sum2 : Sum  Inputs=-|+  OutDataTypeStr=single
  Terminator : Terminator
  theta : Outport  OutDataTypeStr=single
  omega : Outport  Port=2  OutDataTypeStr=single
  SinCos : Outport  Port=3  OutDataTypeStr=single
  wires:
  Product2/1 -> Sum2/1
  Inte_Limit/1(y(k-1)) -> Cos2/1, Cos1/1, theta/1
  Product3/1 -> Sum2/2
  alpha/1 -> Product2/2
  beta/1 -> Product3/1
  Sum2/1 -> PID Controller/1  "PLL_error"
  PID Controller/1 -> omega/1, Inte_Limit/1(x(k))  "Obe_omega"
  Constant1/1 -> Gain/1
  Gain/1 -> Gain2/1
  Constant2/1 -> Gain1/1
  Gain1/1 -> PID Controller/3
  Mux/1 -> SinCos/1
  Cos2/1 -> Mux/1, [Sin]
  Cos1/1 -> [Cos], Mux/2
  Gain2/1 -> PID Controller/2
  [Sin] -> Product2/1
  [Cos] -> Product3/2

== system NFO/Algorithm/SOSOIFO Obe/SOSOIFO ==
  I_alpha_in : Inport
  alpha_in : Inport  Port=2
  I_beta_in : Inport  Port=3
  beta_in : Inport  Port=4
  Add14 : Sum  Inputs=+-  OutDataTypeStr=single
  Add7 : Sum  Inputs=-+  OutDataTypeStr=single
  Gain1 : Gain  Gain=Ls  OutDataTypeStr=single
  Gain2 : Gain  Gain=Ls  OutDataTypeStr=single
  SOSOGI_alpha : Subsystem
  SOSOGI_beta : Subsystem
  Scope : Scope
  Psi_Cos : Outport
  Psi_Sin : Outport  Port=2
  wires:
  Add7/1 -> Psi_Cos/1
  I_alpha_in/1 -> Gain2/1
  I_beta_in/1 -> Gain1/1
  Gain2/1 -> Add7/1
  Gain1/1 -> Add14/2
  Add14/1 -> Psi_Sin/1
  SOSOGI_alpha/2(omegae) -> Scope/1, SOSOGI_beta/1(omega_e)
  SOSOGI_alpha/1(alpha) -> Add7/2
  SOSOGI_beta/1(beta) -> Add14/1
  alpha_in/1 -> SOSOGI_alpha/1(mux_signal)
  beta_in/1 -> SOSOGI_beta/2(mux_signal)

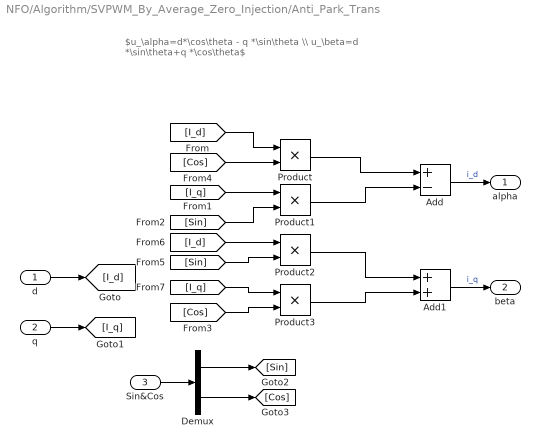
== system NFO/Algorithm/SVPWM_By_Average_Zero_Injection/Anti_Park_Trans ==
  note: $u_\alpha=d*\cos\theta - q *\sin\theta \\ u_\beta=d *\sin\theta+q *\cos\theta$
  d : Inport  OutDataTypeStr=single
  q : Inport  Port=2  OutDataTypeStr=single
  Sin&Cos : Inport  Port=3  OutDataTypeStr=single
  Add : Sum  Inputs=+-  OutDataTypeStr=single
  Add1 : Sum  OutDataTypeStr=single
  Demux : Demux  Outputs=2
  Product{,1..3} (4 alike) : Product  OutDataTypeStr=single
  alpha : Outport  OutDataTypeStr=single
  beta : Outport  Port=2  OutDataTypeStr=single
  wires:
  Add1/1 -> beta/1  "i_q"
  Sin&Cos/1 -> Demux/1
  [Cos] -> Product/2
  Product/1 -> Add/1
  Product1/1 -> Add/2
  q/1 -> [I_q]
  Add/1 -> alpha/1  "i_d"
  [I_d] -> Product/1
  Product3/1 -> Add1/2
  [I_q] -> Product3/1
  [I_q] -> Product1/1
  [Sin] -> Product2/2
  Product2/1 -> Add1/1
  [Sin] -> Product1/2
  [I_d] -> Product2/1
  d/1 -> [I_d]
  [Cos] -> Product3/2
  Demux/1 -> [Sin]
  Demux/2 -> [Cos]

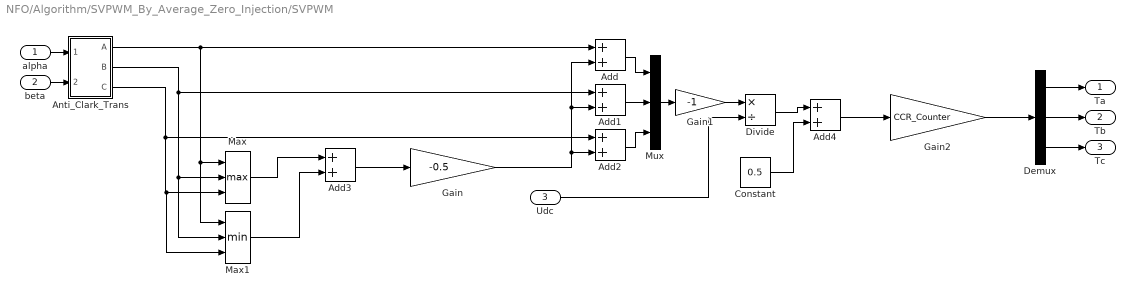
== system NFO/Algorithm/SVPWM_By_Average_Zero_Injection/SVPWM ==
  alpha : Inport  OutDataTypeStr=single
  beta : Inport  Port=2  OutDataTypeStr=single
  Udc : Inport  Port=3  OutDataTypeStr=single
  Add{,1..4} (5 alike) : Sum  OutDataTypeStr=single
  Anti_Clark_Trans : Subsystem
  Constant : Constant  Value=0.5  OutDataTypeStr=single  SampleTime=Ts
  Demux : Demux  Outputs=3
  Divide : Product  Inputs=*/  OutDataTypeStr=single
  Gain : Gain  Gain=-0.5  OutDataTypeStr=single
  Gain1 : Gain  Gain=-1  OutDataTypeStr=single
  Gain2 : Gain  Gain=CCR_Counter  OutDataTypeStr=single
  Max : MinMax  Function=max  Inputs=3  OutDataTypeStr=single
  Max1 : MinMax  Inputs=3  OutDataTypeStr=single
  Mux : Mux  Inputs=3
  Ta : Outport  OutDataTypeStr=single
  Tb : Outport  Port=2  OutDataTypeStr=single
  Tc : Outport  Port=3  OutDataTypeStr=single
  wires:
  Anti_Clark_Trans/1(A) -> Max1/1, Max/1, Add/1
  Gain/1 -> Add/2, Add1/2, Add2/2
  Anti_Clark_Trans/2(B) -> Max1/2, Max/2, Add1/1
  Anti_Clark_Trans/3(C) -> Max1/3, Max/3, Add2/1
  Add3/1 -> Gain/1
  Max/1 -> Add3/1
  alpha/1 -> Anti_Clark_Trans/1(alpha)
  beta/1 -> Anti_Clark_Trans/2(beta)
  Add/1 -> Mux/1
  Add1/1 -> Mux/2
  Add2/1 -> Mux/3
  Demux/1 -> Ta/1
  Demux/2 -> Tb/1
  Demux/3 -> Tc/1
  Divide/1 -> Add4/1
  Constant/1 -> Add4/2
  Max1/1 -> Add3/2
  Udc/1 -> Divide/2
  Add4/1 -> Gain2/1
  Mux/1 -> Gain1/1
  Gain1/1 -> Divide/1
  Gain2/1 -> Demux/1

== system NFO/Algorithm/IF_Gen/IFneg/integrator ==
  note: $y(k)=x(k)*T_s+y(k-1)$
  x(k) : Inport  OutDataTypeStr=single
  RangeLimit : Subsystem
  Sum1 : Sum  Inputs=|++  OutDataTypeStr=single
  Ts : Gain  Gain=Ts  OutDataTypeStr=single
  Unit Delay : UnitDelay  SampleTime=-1  HasFrameUpgradeWarning=on
  y(k-1) : Outport  OutDataTypeStr=single
  wires:
  RangeLimit/1(Theta) -> Unit Delay/1
  Unit Delay/1 -> Sum1/2, y(k-1)/1
  Sum1/1 -> RangeLimit/1(In)  "y(k)"
  Ts/1 -> Sum1/1
  x(k)/1 -> Ts/1

== system NFO/Algorithm/IF_Gen/IFpos/integrator ==
  note: $y(k)=x(k)*T_s+y(k-1)$
  x(k) : Inport  OutDataTypeStr=single
  RangeLimit : Subsystem
  Sum1 : Sum  Inputs=|++  OutDataTypeStr=single
  Ts : Gain  Gain=Ts  OutDataTypeStr=single
  Unit Delay : UnitDelay  SampleTime=-1  HasFrameUpgradeWarning=on
  y(k-1) : Outport  OutDataTypeStr=single
  wires:
  x(k)/1 -> Ts/1
  Ts/1 -> Sum1/1
  Sum1/1 -> RangeLimit/1(In)  "y(k)"
  Unit Delay/1 -> y(k-1)/1, Sum1/2
  RangeLimit/1(Theta) -> Unit Delay/1

== system NFO/Algorithm/SOSOIFO Obe/PLL/Inte_Limit ==
  x(k) : Inport  OutDataTypeStr=single
  Delay : Delay  DelayLength=1
  Sum1 : Sum  Inputs=|++  OutDataTypeStr=single
  Ts : Gain  Gain=Ts  OutDataTypeStr=single
  xianfu : Subsystem
  y(k-1) : Outport  OutDataTypeStr=single
  wires:
  x(k)/1 -> Ts/1
  Ts/1 -> Sum1/1
  Sum1/1 -> xianfu/1(In)
  Delay/1 -> y(k-1)/1, Sum1/2
  xianfu/1(Theta) -> Delay/1

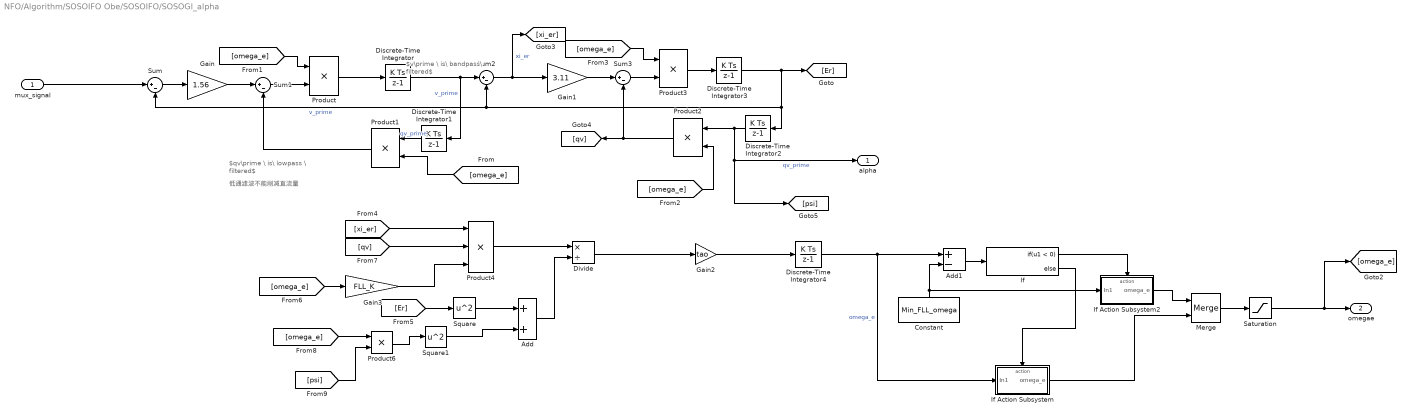
== system NFO/Algorithm/SOSOIFO Obe/SOSOIFO/SOSOGI_alpha ==
  note: $qv\prime \ is\ lowpass \ filtered$
  note: $v\prime \ is\ bandpass\ filtered$
  note: 低通滤波不能削减直流量
  mux_signal : Inport  OutDataTypeStr=single
  Add : Sum
  Add1 : Sum  Inputs=+-  OutDataTypeStr=single
  Constant : Constant  Value=Min_FLL_omega  OutDataTypeStr=single
  Discrete-Time Integrator : DiscreteIntegrator  InitialCondition=1  SampleTime=-1  OutDataTypeStr=single  ICPrevOutput=DiscIntNeverNeededParam  ICPrevScaledInput=DiscIntNeverNeededParam
  Discrete-Time Integrator1 : DiscreteIntegrator  InitialCondition=1  SampleTime=-1  OutDataTypeStr=single  ICPrevOutput=DiscIntNeverNeededParam  ICPrevScaledInput=DiscIntNeverNeededParam
  Discrete-Time Integrator2 : DiscreteIntegrator  InitialCondition=flux  SampleTime=-1  OutDataTypeStr=single  ICPrevOutput=DiscIntNeverNeededParam  ICPrevScaledInput=DiscIntNeverNeededParam
  Discrete-Time Integrator3 : DiscreteIntegrator  InitialCondition=1  SampleTime=-1  OutDataTypeStr=single  ICPrevOutput=DiscIntNeverNeededParam  ICPrevScaledInput=DiscIntNeverNeededParam
  Discrete-Time Integrator4 : DiscreteIntegrator  InitialCondition=200  SampleTime=-1  OutDataTypeStr=single  ICPrevOutput=DiscIntNeverNeededParam  ICPrevScaledInput=DiscIntNeverNeededParam
  Divide : Product  Inputs=*/
  Gain : Gain  Gain=1.56  OutDataTypeStr=single
  Gain1 : Gain  Gain=3.11  OutDataTypeStr=single
  Gain2 : Gain  Gain=tao
  Gain3 : Gain  Gain=FLL_K
  If : If  IfExpression=u1 < 0
  If Action Subsystem : Subsystem  TreatAsAtomicUnit=on
  If Action Subsystem2 : Subsystem  TreatAsAtomicUnit=on
  Merge : Merge
  Product{,1..3} (4 alike) : Product  OutDataTypeStr=single
  Product4 : Product  Inputs=3
  Product6 : Product
  Saturation : Saturate  UpperLimit=1500  LowerLimit=Min_FLL_omega
  Square : Math  Operator=square
  Square1 : Math  Operator=square
  Sum{,1..3} (4 alike) : Sum  Inputs=|+-  OutDataTypeStr=single
  alpha : Outport
  omegae : Outport  Port=2
  wires:
  Product1/1 -> Sum1/2
  Discrete-Time Integrator1/1 -> Product1/1  "qv_prime"
  mux_signal/1 -> Sum/1
  Sum1/1 -> Product/2
  Discrete-Time Integrator/1 -> Sum2/1, Discrete-Time Integrator1/1  "v_prime"
  [omega_e] -> Product/1
  [omega_e] -> Product1/2
  Sum/1 -> Gain/1
  Product/1 -> Discrete-Time Integrator/1
  Gain/1 -> Sum1/1
  Sum2/1 -> [xi_er], Gain1/1  "xi_er"
  Gain1/1 -> Sum3/1
  Discrete-Time Integrator2/1 -> [psi], alpha/1, Product2/1  "qv_prime"
  [omega_e] -> Product2/2
  [omega_e] -> Product3/1
  Sum3/1 -> Product3/2
  Product3/1 -> Discrete-Time Integrator3/1
  Discrete-Time Integrator3/1 -> [Er], Sum2/2, Sum/2, Discrete-Time Integrator2/1  "v_prime"
  Product2/1 -> [qv], Sum3/2
  [xi_er] -> Product4/1
  [Er] -> Square/1
  [omega_e] -> Gain3/1
  Gain3/1 -> Product4/3
  [qv] -> Product4/2
  Product4/1 -> Divide/1
  Square/1 -> Add/1
  [omega_e] -> Product6/1
  [psi] -> Product6/2
  Product6/1 -> Square1/1
  Square1/1 -> Add/2
  Add/1 -> Divide/2
  Add1/1 -> If/1
  Discrete-Time Integrator4/1 -> If Action Subsystem/1(In1), Add1/1  "omega_e"
  Constant/1 -> If Action Subsystem2/1(In1), Add1/2
  If Action Subsystem2/1(omega_e) -> Merge/1
  If Action Subsystem/1(omega_e) -> Merge/2
  If/1 -> If Action Subsystem2/Action
  If/2 -> If Action Subsystem/Action
  Merge/1 -> Saturation/1
  Divide/1 -> Gain2/1
  Saturation/1 -> [omega_e], omegae/1
  Gain2/1 -> Discrete-Time Integrator4/1

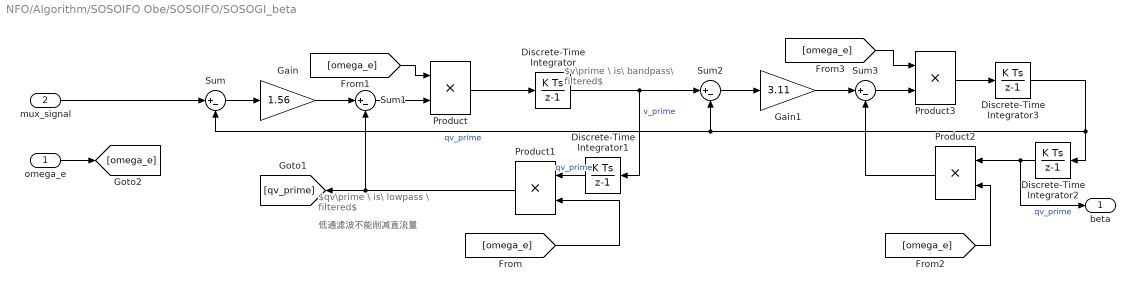
== system NFO/Algorithm/SOSOIFO Obe/SOSOIFO/SOSOGI_beta ==
  note: 低通滤波不能削减直流量
  note: $v\prime \ is\ bandpass\ filtered$
  note: $qv\prime \ is\ lowpass \ filtered$
  omega_e : Inport  OutDataTypeStr=single
  mux_signal : Inport  Port=2  OutDataTypeStr=single
  Discrete-Time Integrator : DiscreteIntegrator  InitialCondition=1  SampleTime=-1  OutDataTypeStr=single  ICPrevOutput=DiscIntNeverNeededParam  ICPrevScaledInput=DiscIntNeverNeededParam
  Discrete-Time Integrator1 : DiscreteIntegrator  InitialCondition=1  SampleTime=-1  OutDataTypeStr=single  ICPrevOutput=DiscIntNeverNeededParam  ICPrevScaledInput=DiscIntNeverNeededParam
  Discrete-Time Integrator2 : DiscreteIntegrator  InitialCondition=flux  SampleTime=-1  OutDataTypeStr=single  ICPrevOutput=DiscIntNeverNeededParam  ICPrevScaledInput=DiscIntNeverNeededParam
  Discrete-Time Integrator3 : DiscreteIntegrator  InitialCondition=1  SampleTime=-1  OutDataTypeStr=single  ICPrevOutput=DiscIntNeverNeededParam  ICPrevScaledInput=DiscIntNeverNeededParam
  Gain : Gain  Gain=1.56  OutDataTypeStr=single
  Gain1 : Gain  Gain=3.11  OutDataTypeStr=single
  Product{,1..3} (4 alike) : Product  OutDataTypeStr=single
  Sum{,1..3} (4 alike) : Sum  Inputs=|+-  OutDataTypeStr=single
  beta : Outport
  wires:
  Product2/1 -> Sum3/2
  Discrete-Time Integrator3/1 -> Discrete-Time Integrator2/1, Sum/2, Sum2/2  "qv_prime"
  Product3/1 -> Discrete-Time Integrator3/1
  Sum3/1 -> Product3/2
  [omega_e] -> Product3/1
  [omega_e] -> Product2/2
  Discrete-Time Integrator2/1 -> Product2/1, beta/1  "qv_prime"
  Gain1/1 -> Sum3/1
  Sum2/1 -> Gain1/1
  Gain/1 -> Sum1/1
  Product/1 -> Discrete-Time Integrator/1
  Sum/1 -> Gain/1
  [omega_e] -> Product1/2
  [omega_e] -> Product/1
  Discrete-Time Integrator/1 -> Discrete-Time Integrator1/1, Sum2/1  "v_prime"
  Sum1/1 -> Product/2
  mux_signal/1 -> Sum/1
  omega_e/1 -> [omega_e]
  Discrete-Time Integrator1/1 -> Product1/1  "qv_prime"
  Product1/1 -> Sum1/2, [qv_prime]

== system NFO/Algorithm/SVPWM_By_Average_Zero_Injection/SVPWM/Anti_Clark_Trans ==
  alpha : Inport  OutDataTypeStr=single
  beta : Inport  Port=2  OutDataTypeStr=single
  Add : Sum  Inputs=-+  OutDataTypeStr=single
  Add1 : Sum  Inputs=--  OutDataTypeStr=single
  Gain : Gain  Gain=0.5  OutDataTypeStr=single
  Gain1 : Gain  Gain=sqrt(3)/2  OutDataTypeStr=single
  A : Outport  OutDataTypeStr=single
  B : Outport  Port=2  OutDataTypeStr=single
  C : Outport  Port=3  OutDataTypeStr=single
  wires:
  Add1/1 -> C/1
  Gain/1 -> Add1/1, Add/1
  Add/1 -> B/1
  alpha/1 -> A/1, Gain/1
  Gain1/1 -> Add1/2, Add/2
  beta/1 -> Gain1/1

== system NFO/Algorithm/IF_Gen/IFneg/integrator/RangeLimit ==
  In : Inport  OutDataTypeStr=single
  Constant : Constant  Value=2*pi  OutDataTypeStr=single  SampleTime=-1
  Constant1 : Constant  Value=0  OutDataTypeStr=single  SampleTime=-1
  If : If  NumInputs=2  IfExpression=u1  ElseIfExpressions=u2
  If Action Subsystem : Subsystem  TreatAsAtomicUnit=on
  If Action Subsystem1 : Subsystem  TreatAsAtomicUnit=on
  If Action Subsystem2 : Subsystem  TreatAsAtomicUnit=on
  Merge : Merge  Inputs=3
  Relational Operator : RelationalOperator  Operator=>  OutDataTypeStr=boolean  RndMeth=Simplest  InputSameDT=off
  Relational Operator1 : RelationalOperator  Operator=<  OutDataTypeStr=boolean  RndMeth=Simplest  InputSameDT=off
  Theta : Outport  OutDataTypeStr=single
  wires:
  If Action Subsystem1/1(Out1) -> Merge/3
  If Action Subsystem/1(Out1) -> Merge/2
  If Action Subsystem2/1(Out1) -> Merge/1
  If/1 -> If Action Subsystem1/Action
  If/2 -> If Action Subsystem/Action
  If/3 -> If Action Subsystem2/Action
  Merge/1 -> Theta/1
  Relational Operator1/1 -> If/2
  In/1 -> Relational Operator/1, If Action Subsystem/1(In1), If Action Subsystem1/1(In1), If Action Subsystem2/1(In1), Relational Operator1/1
  Constant1/1 -> Relational Operator1/2
  Constant/1 -> Relational Operator/2
  Relational Operator/1 -> If/1
